simulink model "untitled"  (R2018a)
settings: Solver=FixedStepDiscrete  StartTime=0.0  StopTime=100  RelTol=1e-3
values from neighbouring files (symbols this model uses):
  coeff = randi([0, 1], 3, 60)*2-1    [Untitled.m]
libraries: filter_library x261, simulink x2, dspsrcs4 x1
(part 2 of 2)

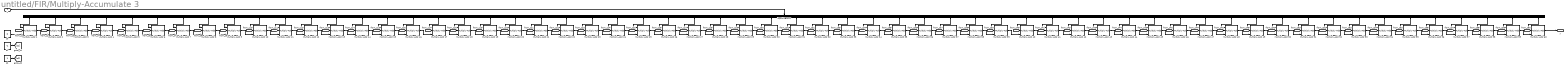
== system untitled/FIR/Multiply-Accumulate 3 ==
  x : Inport
  Input Demux : Demux  Outputs=60
  Multiply-Add {1..60} (60 alike) : filter_library/Multiply-Add  SystemSampleTime=-1
      settings: SourceProductName=Filter Library
  c0 : Constant  Value=0  OutDataTypeStr=fixdt(1, 12, 7)  SampleTime=1
  c1 : Constant  Value=-1  OutDataTypeStr=fixdt(1, 12, 7)  SampleTime=1
  c2 : Constant  OutDataTypeStr=fixdt(1, 12, 7)  SampleTime=1
  y : Outport
  wires:
  [c2] -> Multiply-Add 1/2
  [c1] -> Multiply-Add 2/2
  [c2] -> Multiply-Add 3/2
  [c2] -> Multiply-Add 4/2
  [c1] -> Multiply-Add 5/2
  [c1] -> Multiply-Add 6/2
  [c1] -> Multiply-Add 7/2
  [c2] -> Multiply-Add 8/2
  [c2] -> Multiply-Add 9/2
  [c2] -> Multiply-Add 10/2
  [c1] -> Multiply-Add 11/2
  [c1] -> Multiply-Add 12/2
  [c1] -> Multiply-Add 13/2
  [c2] -> Multiply-Add 14/2
  [c2] -> Multiply-Add 15/2
  [c2] -> Multiply-Add 16/2
  [c2] -> Multiply-Add 17/2
  [c2] -> Multiply-Add 18/2
  [c2] -> Multiply-Add 19/2
  [c1] -> Multiply-Add 20/2
  [c1] -> Multiply-Add 21/2
  [c1] -> Multiply-Add 22/2
  [c2] -> Multiply-Add 23/2
  [c2] -> Multiply-Add 24/2
  [c2] -> Multiply-Add 25/2
  [c2] -> Multiply-Add 26/2
  [c1] -> Multiply-Add 27/2
  [c2] -> Multiply-Add 28/2
  [c1] -> Multiply-Add 29/2
  [c2] -> Multiply-Add 30/2
  [c2] -> Multiply-Add 31/2
  [c1] -> Multiply-Add 32/2
  [c2] -> Multiply-Add 33/2
  [c2] -> Multiply-Add 34/2
  [c1] -> Multiply-Add 35/2
  [c2] -> Multiply-Add 36/2
  [c2] -> Multiply-Add 37/2
  [c2] -> Multiply-Add 38/2
  [c2] -> Multiply-Add 39/2
  [c1] -> Multiply-Add 40/2
  [c1] -> Multiply-Add 41/2
  [c1] -> Multiply-Add 42/2
  [c1] -> Multiply-Add 43/2
  [c2] -> Multiply-Add 44/2
  [c1] -> Multiply-Add 45/2
  [c2] -> Multiply-Add 46/2
  [c2] -> Multiply-Add 47/2
  [c2] -> Multiply-Add 48/2
  [c2] -> Multiply-Add 49/2
  [c1] -> Multiply-Add 50/2
  [c1] -> Multiply-Add 51/2
  [c1] -> Multiply-Add 52/2
  [c2] -> Multiply-Add 53/2
  [c2] -> Multiply-Add 54/2
  [c1] -> Multiply-Add 55/2
  [c1] -> Multiply-Add 56/2
  [c1] -> Multiply-Add 57/2
  [c2] -> Multiply-Add 58/2
  [c1] -> Multiply-Add 59/2
  [c2] -> Multiply-Add 60/2
  Multiply-Add 1/1 -> Multiply-Add 2/3
  Multiply-Add 2/1 -> Multiply-Add 3/3
  Multiply-Add 3/1 -> Multiply-Add 4/3
  Multiply-Add 4/1 -> Multiply-Add 5/3
  Multiply-Add 5/1 -> Multiply-Add 6/3
  Multiply-Add 6/1 -> Multiply-Add 7/3
  Multiply-Add 7/1 -> Multiply-Add 8/3
  Multiply-Add 8/1 -> Multiply-Add 9/3
  Multiply-Add 9/1 -> Multiply-Add 10/3
  Multiply-Add 10/1 -> Multiply-Add 11/3
  Multiply-Add 11/1 -> Multiply-Add 12/3
  Multiply-Add 12/1 -> Multiply-Add 13/3
  Multiply-Add 13/1 -> Multiply-Add 14/3
  Multiply-Add 14/1 -> Multiply-Add 15/3
  Multiply-Add 15/1 -> Multiply-Add 16/3
  Multiply-Add 16/1 -> Multiply-Add 17/3
  Multiply-Add 17/1 -> Multiply-Add 18/3
  Multiply-Add 18/1 -> Multiply-Add 19/3
  Multiply-Add 19/1 -> Multiply-Add 20/3
  Multiply-Add 20/1 -> Multiply-Add 21/3
  Multiply-Add 21/1 -> Multiply-Add 22/3
  Multiply-Add 22/1 -> Multiply-Add 23/3
  Multiply-Add 23/1 -> Multiply-Add 24/3
  Multiply-Add 24/1 -> Multiply-Add 25/3
  Multiply-Add 25/1 -> Multiply-Add 26/3
  Multiply-Add 26/1 -> Multiply-Add 27/3
  Multiply-Add 27/1 -> Multiply-Add 28/3
  Multiply-Add 28/1 -> Multiply-Add 29/3
  Multiply-Add 29/1 -> Multiply-Add 30/3
  Multiply-Add 30/1 -> Multiply-Add 31/3
  Multiply-Add 31/1 -> Multiply-Add 32/3
  Multiply-Add 32/1 -> Multiply-Add 33/3
  Multiply-Add 33/1 -> Multiply-Add 34/3
  Multiply-Add 34/1 -> Multiply-Add 35/3
  Multiply-Add 35/1 -> Multiply-Add 36/3
  Multiply-Add 36/1 -> Multiply-Add 37/3
  Multiply-Add 37/1 -> Multiply-Add 38/3
  Multiply-Add 38/1 -> Multiply-Add 39/3
  Multiply-Add 39/1 -> Multiply-Add 40/3
  Multiply-Add 40/1 -> Multiply-Add 41/3
  Multiply-Add 41/1 -> Multiply-Add 42/3
  Multiply-Add 42/1 -> Multiply-Add 43/3
  Multiply-Add 43/1 -> Multiply-Add 44/3
  Multiply-Add 44/1 -> Multiply-Add 45/3
  Multiply-Add 45/1 -> Multiply-Add 46/3
  Multiply-Add 46/1 -> Multiply-Add 47/3
  Multiply-Add 47/1 -> Multiply-Add 48/3
  Multiply-Add 48/1 -> Multiply-Add 49/3
  Multiply-Add 49/1 -> Multiply-Add 50/3
  Multiply-Add 50/1 -> Multiply-Add 51/3
  Multiply-Add 51/1 -> Multiply-Add 52/3
  Multiply-Add 52/1 -> Multiply-Add 53/3
  Multiply-Add 53/1 -> Multiply-Add 54/3
  Multiply-Add 54/1 -> Multiply-Add 55/3
  Multiply-Add 55/1 -> Multiply-Add 56/3
  Multiply-Add 56/1 -> Multiply-Add 57/3
  Multiply-Add 57/1 -> Multiply-Add 58/3
  Multiply-Add 58/1 -> Multiply-Add 59/3
  Multiply-Add 59/1 -> Multiply-Add 60/3
  Multiply-Add 60/1 -> y/1
  x/1 -> Input Demux/1
  Input Demux/1 -> Multiply-Add 1/1
  Input Demux/2 -> Multiply-Add 2/1
  Input Demux/3 -> Multiply-Add 3/1
  Input Demux/4 -> Multiply-Add 4/1
  Input Demux/5 -> Multiply-Add 5/1
  Input Demux/6 -> Multiply-Add 6/1
  Input Demux/7 -> Multiply-Add 7/1
  Input Demux/8 -> Multiply-Add 8/1
  Input Demux/9 -> Multiply-Add 9/1
  Input Demux/10 -> Multiply-Add 10/1
  Input Demux/11 -> Multiply-Add 11/1
  Input Demux/12 -> Multiply-Add 12/1
  Input Demux/13 -> Multiply-Add 13/1
  Input Demux/14 -> Multiply-Add 14/1
  Input Demux/15 -> Multiply-Add 15/1
  Input Demux/16 -> Multiply-Add 16/1
  Input Demux/17 -> Multiply-Add 17/1
  Input Demux/18 -> Multiply-Add 18/1
  Input Demux/19 -> Multiply-Add 19/1
  Input Demux/20 -> Multiply-Add 20/1
  Input Demux/21 -> Multiply-Add 21/1
  Input Demux/22 -> Multiply-Add 22/1
  Input Demux/23 -> Multiply-Add 23/1
  Input Demux/24 -> Multiply-Add 24/1
  Input Demux/25 -> Multiply-Add 25/1
  Input Demux/26 -> Multiply-Add 26/1
  Input Demux/27 -> Multiply-Add 27/1
  Input Demux/28 -> Multiply-Add 28/1
  Input Demux/29 -> Multiply-Add 29/1
  Input Demux/30 -> Multiply-Add 30/1
  Input Demux/31 -> Multiply-Add 31/1
  Input Demux/32 -> Multiply-Add 32/1
  Input Demux/33 -> Multiply-Add 33/1
  Input Demux/34 -> Multiply-Add 34/1
  Input Demux/35 -> Multiply-Add 35/1
  Input Demux/36 -> Multiply-Add 36/1
  Input Demux/37 -> Multiply-Add 37/1
  Input Demux/38 -> Multiply-Add 38/1
  Input Demux/39 -> Multiply-Add 39/1
  Input Demux/40 -> Multiply-Add 40/1
  Input Demux/41 -> Multiply-Add 41/1
  Input Demux/42 -> Multiply-Add 42/1
  Input Demux/43 -> Multiply-Add 43/1
  Input Demux/44 -> Multiply-Add 44/1
  Input Demux/45 -> Multiply-Add 45/1
  Input Demux/46 -> Multiply-Add 46/1
  Input Demux/47 -> Multiply-Add 47/1
  Input Demux/48 -> Multiply-Add 48/1
  Input Demux/49 -> Multiply-Add 49/1
  Input Demux/50 -> Multiply-Add 50/1
  Input Demux/51 -> Multiply-Add 51/1
  Input Demux/52 -> Multiply-Add 52/1
  Input Demux/53 -> Multiply-Add 53/1
  Input Demux/54 -> Multiply-Add 54/1
  Input Demux/55 -> Multiply-Add 55/1
  Input Demux/56 -> Multiply-Add 56/1
  Input Demux/57 -> Multiply-Add 57/1
  Input Demux/58 -> Multiply-Add 58/1
  Input Demux/59 -> Multiply-Add 59/1
  Input Demux/60 -> Multiply-Add 60/1
  c1/1 -> [c1]
  c2/1 -> [c2]
  c0/1 -> Multiply-Add 1/3
